simulink model "HLB_LDMPoly_cpp"  (R2019b)
settings: Solver=FixedStepDiscrete  StartTime=0.0  StopTime=10.0  FixedStep=0.01  RelTol=1e-3
settings Model: Creator=IGG2BP  LastModifiedBy=DOT1BP
settings ModelReferenceCC: ModelReferenceNumInstancesAllowed=Single

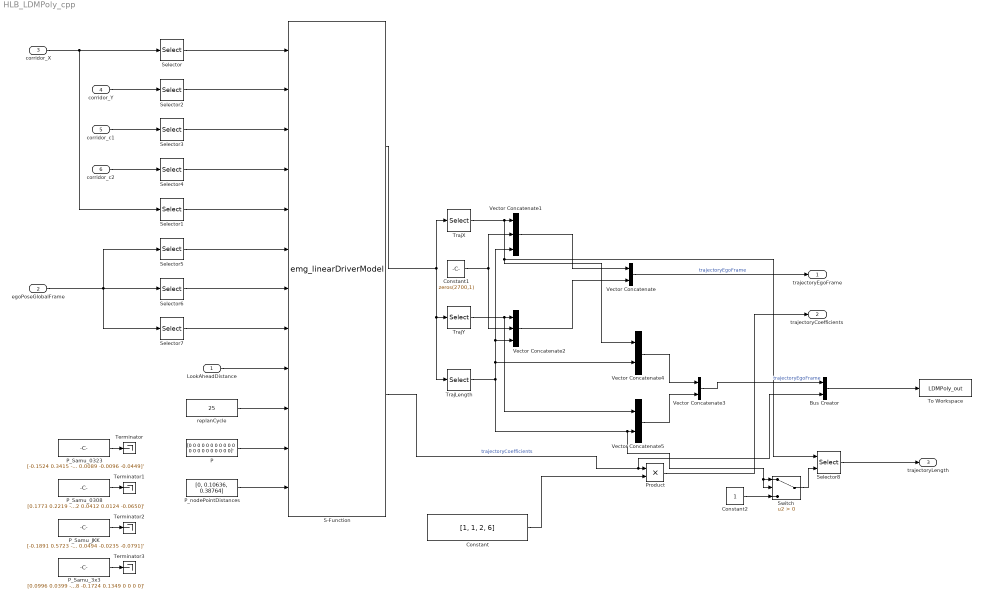
== system HLB_LDMPoly_cpp ==
  LookAheadDistance : Inport
  egoPoseGlobalFrame : Inport  Port=2
  corridor_X : Inport  Port=3
  corridor_Y : Inport  Port=4
  corridor_c1 : Inport  Port=5
  corridor_c2 : Inport  Port=6
  Bus Creator : BusCreator  Inputs=2
  Constant : Constant  Value=[1, 1, 2, 6]
  Constant1 : Constant  Value=zeros(2700,1)
  Constant2 : Constant
  P : Constant  Value=[0 0 0 0 0 0 0 0 0 0 0 0 0 0 0 0 0 0 0 0 0]'
  P_Samu_0308 : Constant  Value=[0.1773 0.2219 -0.2682 -0.0332 0.0887 0.0013 0.0761 -0.3368 0.7714 -0.3123 0.0194 -0.0027 0.0293 0.0384 0.2913 -0.4504 0.2953 -0.0362 0.0412 0.0124 -0.0650]'
  P_Samu_0323 : Constant  Value=[-0.1524 0.3415 -0.1253 -0.0464 0.0239 -0.0055 0.0215 0.1143 0.0686 -0.1218 -0.0161 0.0354 0.0297 -0.0039 0.3901 -0.5318 0.2184 0.0146 0.0089 -0.0096 -0.0449]'
  P_Samu_3x3 : Constant  Value=[0.0996 0.0399 -0.0811 0 0 0 0 -0.0754 0.2313 -0.0940 0 0 0 0 0.1228 -0.1724 0.1349 0 0 0 0]'
  P_Samu_JKK : Constant  Value=[-0.1891 0.5723 -0.2526 -0.0105 0.0167 -0.0250 0.0681 -0.4980 0.9711 -0.3461 0.0010 -0.0047 0.0333 0.0391 0.6295 -0.8867 0.3919 0.0183 0.0494 -0.0235 -0.0791]'
  P_nodePointDistances : Constant  Value=[0, 0.10636, 0.38764]
  Product : Product
  S-Function : S-Function  FunctionName=emg_linearDriverModel  SFunctionDeploymentMode=off  EnableBusSupport=off
  Selector{,2..4} (4 alike) : Selector  InputPortWidth=301  IndexOptions=Index vector (dialog)  Indices=linspace(1,300,300)  OutputSizes=1
  Selector1 : Selector  InputPortWidth=301  IndexOptions=Index vector (dialog)  Indices=301  OutputSizes=1
  Selector5 : Selector  InputPortWidth=3  IndexOptions=Index vector (dialog)  Indices=1  OutputSizes=1
  Selector6 : Selector  InputPortWidth=3  IndexOptions=Index vector (dialog)  Indices=2  OutputSizes=1
  Selector7 : Selector  InputPortWidth=3  IndexOptions=Index vector (dialog)  Indices=3  OutputSizes=1
  Selector8 : Selector  InputPortWidth=300  IndexOptions=Index vector (port)  Indices=[1 3]  OutputSizes=1
  Switch : Switch  Criteria=u2 > Threshold
  Terminator{,1..3} (4 alike) : Terminator
  To Workspace : ToWorkspace  VariableName=LDMPoly_out  SaveFormat=Timeseries  SampleTime=-1
  TrajLength : Selector  InputPortWidth=601  IndexOptions=Index vector (dialog)  Indices=601  OutputSizes=1
  TrajX : Selector  InputPortWidth=601  IndexOptions=Index vector (dialog)  Indices=linspace(1,300,300)  OutputSizes=1
  TrajY : Selector  InputPortWidth=601  IndexOptions=Index vector (dialog)  Indices=linspace(301,600,300)  OutputSizes=1
  Vector Concatenate : Concatenate  Mode=Multidimensional array  ConcatenateDimension=2
  Vector Concatenate1 : Concatenate  NumInputs=3
  Vector Concatenate2 : Concatenate  NumInputs=3
  Vector Concatenate3 : Concatenate  Mode=Multidimensional array  ConcatenateDimension=2
  Vector Concatenate4 : Concatenate
  Vector Concatenate5 : Concatenate
  replanCycle : Constant  Value=25
  trajectoryEgoFrame : Outport
  trajectoryCoefficients : Outport  Port=2
  trajectoryLength : Outport  Port=3
  wires:
  Bus Creator/1 -> To Workspace/1
  corridor_Y/1 -> Selector2/1
  S-Function/1 -> TrajY/1, TrajLength/1, TrajX/1
  egoPoseGlobalFrame/1 -> Selector7/1, Selector6/1, Selector5/1
  Vector Concatenate1/1 -> Vector Concatenate/1
  TrajX/1 -> Vector Concatenate4/1, Selector8/1, Vector Concatenate1/1
  P_Samu_JKK/1 -> Terminator2/1
  P_Samu_0308/1 -> Terminator1/1
  Vector Concatenate4/1 -> Vector Concatenate3/1
  Selector7/1 -> S-Function/8
  TrajLength/1 -> Vector Concatenate2/3, Vector Concatenate1/3, Vector Concatenate4/2, Switch/1, Switch/2, Vector Concatenate5/2
  TrajY/1 -> Vector Concatenate5/1, Vector Concatenate2/1
  Vector Concatenate5/1 -> Vector Concatenate3/2
  Vector Concatenate2/1 -> Vector Concatenate/2
  Selector5/1 -> S-Function/6
  Selector4/1 -> S-Function/4
  P_Samu_0323/1 -> Terminator/1
  Vector Concatenate3/1 -> Bus Creator/1  "trajectoryEgoFrame"
  Selector3/1 -> S-Function/3
  corridor_c2/1 -> Selector4/1
  Selector2/1 -> S-Function/2
  P_nodePointDistances/1 -> S-Function/12
  Constant1/1 -> Vector Concatenate2/2, Vector Concatenate1/2
  corridor_c1/1 -> Selector3/1
  Selector6/1 -> S-Function/7
  corridor_X/1 -> Selector/1, Selector1/1
  replanCycle/1 -> S-Function/10
  Selector/1 -> S-Function/1
  Selector1/1 -> S-Function/5
  P/1 -> S-Function/11
  LookAheadDistance/1 -> S-Function/9
  S-Function/2 -> Bus Creator/2, Product/1  "trajectoryCoefficients"
  Vector Concatenate/1 -> trajectoryEgoFrame/1  "trajectoryEgoFrame"
  P_Samu_3x3/1 -> Terminator3/1
  Constant/1 -> Product/2
  Product/1 -> trajectoryCoefficients/1
  Selector8/1 -> trajectoryLength/1
  Constant2/1 -> Switch/3
  Switch/1 -> Selector8/2
